simulink model "AttitudeControl"  (R2023a)
settings: Solver=VariableStepAuto  StartTime=0.0  StopTime=10.0  RelTol=1e-3
settings Model: Creator=aan18022  LastModifiedBy=aan18022

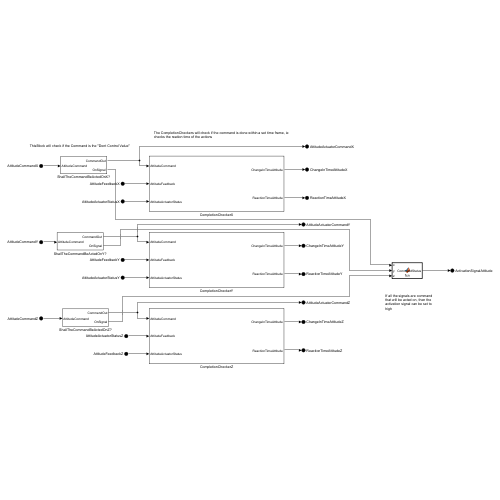
[thumbnail: Simulink's stored preview of the top-level diagram]
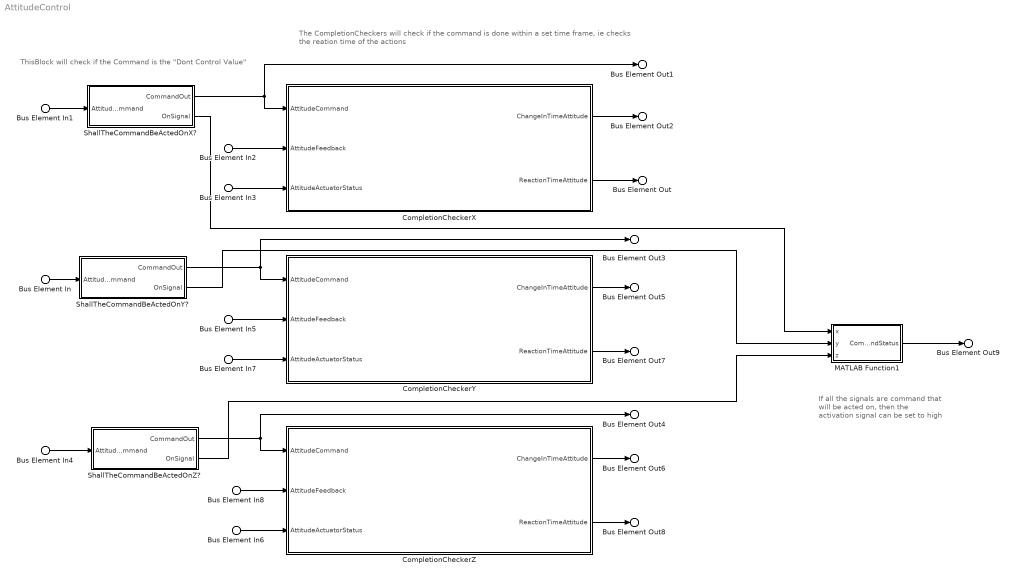
== system AttitudeControl ==
  note: If all the signals are command that will be acted on, then the activation signal can be set to high
  note: The CompletionCheckers will check if the command is done within a set time frame, ie checks the reation time of the actions
  note: ThisBlock will check if the Command is the "Dont Control Value"
  Bus Element In1 : Inport  PortName=AttitudeCommandX
  Bus Element In2 : Inport  Port=2  PortName=AttitudeFeedbackX
  Bus Element In3 : Inport  Port=3  PortName=AttitudeActuatorStatusX
  Bus Element In : Inport  Port=4  PortName=AttitudeCommandY
  Bus Element In4 : Inport  Port=5  PortName=AttitudeCommandZ
  Bus Element In5 : Inport  Port=6  PortName=AttitudeFeedbackY
  Bus Element In6 : Inport  Port=7  PortName=AttitudeFeedbackZ
  Bus Element In7 : Inport  Port=8  PortName=AttitudeActuatorStatusY
  Bus Element In8 : Inport  Port=9  PortName=AttitudeActuatorStatusZ
  CompletionCheckerX : Subsystem
  CompletionCheckerY : Subsystem
  CompletionCheckerZ : Subsystem
  MATLAB Function1 : MATLAB Function  TreatAsAtomicUnit=on
  ShallTheCommandBeActedOnX? : Subsystem
  ShallTheCommandBeActedOnY? : Subsystem
  ShallTheCommandBeActedOnZ? : Subsystem
  Bus Element Out1 : Outport  PortName=AttitudeActuatorCommandX
  Bus Element Out2 : Outport  Port=2  PortName=ChangeInTimeAttitudeX
  Bus Element Out : Outport  Port=3  PortName=ReactionTimeAttitudeX
  Bus Element Out3 : Outport  Port=4  PortName=AttitudeActuatorCommandY
  Bus Element Out4 : Outport  Port=5  PortName=AttitudeActuatorCommandZ
  Bus Element Out5 : Outport  Port=6  PortName=ChangeInTimeAttitudeY
  Bus Element Out6 : Outport  Port=7  PortName=ChangeInTimeAttitudeZ
  Bus Element Out7 : Outport  Port=8  PortName=ReactionTimeAttitudeY
  Bus Element Out8 : Outport  Port=9  PortName=ReactionTimeAttitudeZ
  Bus Element Out9 : Outport  Port=10  PortName=ActivationSignalAttitude
  wires:
  Bus Element In1/1 -> ShallTheCommandBeActedOnX?/1(AttitudeCommand)
  CompletionCheckerY/1(ChangeInTimeAttitude) -> Bus Element Out5/1
  CompletionCheckerY/2(ReactionTimeAttitude) -> Bus Element Out7/1
  Bus Element In2/1 -> CompletionCheckerX/2(AttitudeFeedback)
  Bus Element In8/1 -> CompletionCheckerZ/2(AttitudeFeedback)
  CompletionCheckerZ/2(ReactionTimeAttitude) -> Bus Element Out8/1
  CompletionCheckerX/2(ReactionTimeAttitude) -> Bus Element Out/1
  Bus Element In5/1 -> CompletionCheckerY/2(AttitudeFeedback)
  Bus Element In/1 -> ShallTheCommandBeActedOnY?/1(AttitudeCommand)
  Bus Element In6/1 -> CompletionCheckerZ/3(AttitudeActuatorStatus)
  Bus Element In3/1 -> CompletionCheckerX/3(AttitudeActuatorStatus)
  CompletionCheckerX/1(ChangeInTimeAttitude) -> Bus Element Out2/1
  CompletionCheckerZ/1(ChangeInTimeAttitude) -> Bus Element Out6/1
  Bus Element In4/1 -> ShallTheCommandBeActedOnZ?/1(AttitudeCommand)
  ShallTheCommandBeActedOnX?/1(CommandOut) -> CompletionCheckerX/1(AttitudeCommand), Bus Element Out1/1
  ShallTheCommandBeActedOnY?/1(CommandOut) -> CompletionCheckerY/1(AttitudeCommand), Bus Element Out3/1
  ShallTheCommandBeActedOnZ?/1(CommandOut) -> CompletionCheckerZ/1(AttitudeCommand), Bus Element Out4/1
  Bus Element In7/1 -> CompletionCheckerY/3(AttitudeActuatorStatus)
  ShallTheCommandBeActedOnX?/2(OnSignal) -> MATLAB Function1/1(x)
  ShallTheCommandBeActedOnY?/2(OnSignal) -> MATLAB Function1/2(y)
  ShallTheCommandBeActedOnZ?/2(OnSignal) -> MATLAB Function1/3(z)
  MATLAB Function1/1(CommandStatus) -> Bus Element Out9/1

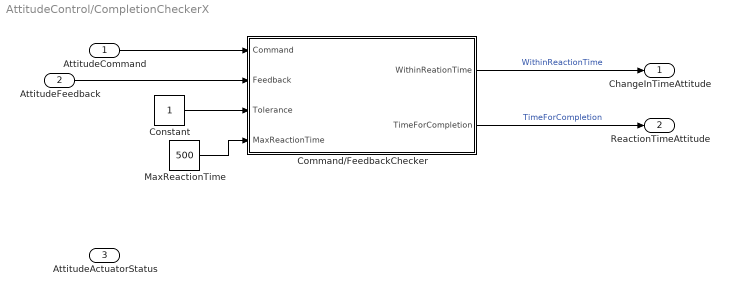
== system AttitudeControl/CompletionCheckerX ==
  AttitudeCommand : Inport
  AttitudeFeedback : Inport  Port=2
  AttitudeActuatorStatus : Inport  Port=3
  Command/FeedbackChecker : Subsystem
  Constant : Constant
  MaxReactionTime : Constant  Value=500
  ChangeInTimeAttitude : Outport
  ReactionTimeAttitude : Outport  Port=2
  wires:
  AttitudeCommand/1 -> Command/FeedbackChecker/1(Command)
  AttitudeFeedback/1 -> Command/FeedbackChecker/2(Feedback)
  Constant/1 -> Command/FeedbackChecker/3(Tolerance)
  Command/FeedbackChecker/1(WithinReationTime) -> ChangeInTimeAttitude/1  "WithinReactionTime"
  Command/FeedbackChecker/2(TimeForCompletion) -> ReactionTimeAttitude/1  "TimeForCompletion"
  MaxReactionTime/1 -> Command/FeedbackChecker/4(MaxReactionTime)

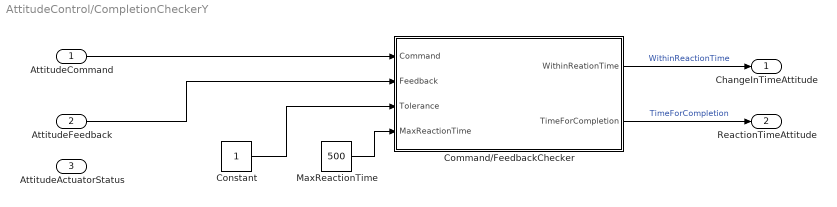
== system AttitudeControl/CompletionCheckerY ==
  AttitudeCommand : Inport
  AttitudeFeedback : Inport  Port=2
  AttitudeActuatorStatus : Inport  Port=3
  Command/FeedbackChecker : Subsystem
  Constant : Constant
  MaxReactionTime : Constant  Value=500
  ChangeInTimeAttitude : Outport
  ReactionTimeAttitude : Outport  Port=2
  wires:
  AttitudeCommand/1 -> Command/FeedbackChecker/1(Command)
  AttitudeFeedback/1 -> Command/FeedbackChecker/2(Feedback)
  Constant/1 -> Command/FeedbackChecker/3(Tolerance)
  Command/FeedbackChecker/1(WithinReationTime) -> ChangeInTimeAttitude/1  "WithinReactionTime"
  Command/FeedbackChecker/2(TimeForCompletion) -> ReactionTimeAttitude/1  "TimeForCompletion"
  MaxReactionTime/1 -> Command/FeedbackChecker/4(MaxReactionTime)

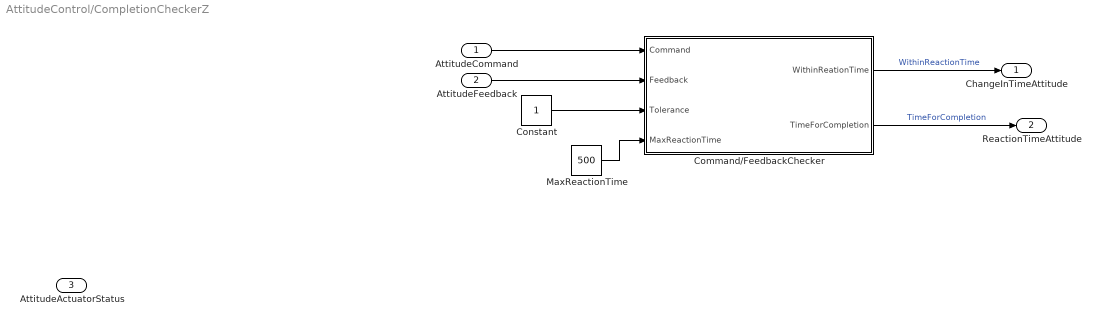
== system AttitudeControl/CompletionCheckerZ ==
  AttitudeCommand : Inport
  AttitudeFeedback : Inport  Port=2
  AttitudeActuatorStatus : Inport  Port=3
  Command/FeedbackChecker : Subsystem
  Constant : Constant
  MaxReactionTime : Constant  Value=500
  ChangeInTimeAttitude : Outport
  ReactionTimeAttitude : Outport  Port=2
  wires:
  AttitudeCommand/1 -> Command/FeedbackChecker/1(Command)
  AttitudeFeedback/1 -> Command/FeedbackChecker/2(Feedback)
  Constant/1 -> Command/FeedbackChecker/3(Tolerance)
  Command/FeedbackChecker/1(WithinReationTime) -> ChangeInTimeAttitude/1  "WithinReactionTime"
  Command/FeedbackChecker/2(TimeForCompletion) -> ReactionTimeAttitude/1  "TimeForCompletion"
  MaxReactionTime/1 -> Command/FeedbackChecker/4(MaxReactionTime)

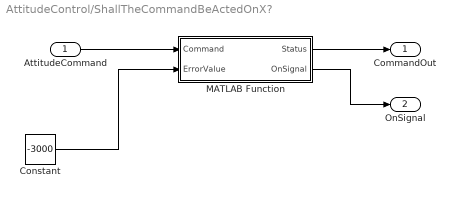
== system AttitudeControl/ShallTheCommandBeActedOnX? ==
  AttitudeCommand : Inport
  Constant : Constant  Value=-3000
  MATLAB Function : MATLAB Function  TreatAsAtomicUnit=on
  CommandOut : Outport
  OnSignal : Outport  Port=2
  wires:
  Constant/1 -> MATLAB Function/2(ErrorValue)
  AttitudeCommand/1 -> MATLAB Function/1(Command)
  MATLAB Function/1(Status) -> CommandOut/1
  MATLAB Function/2(OnSignal) -> OnSignal/1

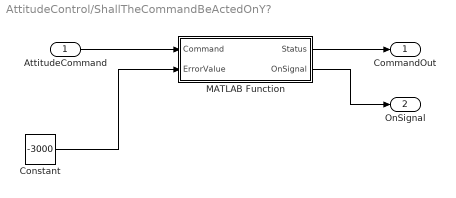
== system AttitudeControl/ShallTheCommandBeActedOnY? ==
  AttitudeCommand : Inport
  Constant : Constant  Value=-3000
  MATLAB Function : MATLAB Function  TreatAsAtomicUnit=on
  CommandOut : Outport
  OnSignal : Outport  Port=2
  wires:
  Constant/1 -> MATLAB Function/2(ErrorValue)
  AttitudeCommand/1 -> MATLAB Function/1(Command)
  MATLAB Function/1(Status) -> CommandOut/1
  MATLAB Function/2(OnSignal) -> OnSignal/1

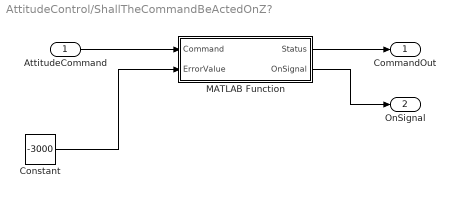
== system AttitudeControl/ShallTheCommandBeActedOnZ? ==
  AttitudeCommand : Inport
  Constant : Constant  Value=-3000
  MATLAB Function : MATLAB Function  TreatAsAtomicUnit=on
  CommandOut : Outport
  OnSignal : Outport  Port=2
  wires:
  Constant/1 -> MATLAB Function/2(ErrorValue)
  AttitudeCommand/1 -> MATLAB Function/1(Command)
  MATLAB Function/1(Status) -> CommandOut/1
  MATLAB Function/2(OnSignal) -> OnSignal/1

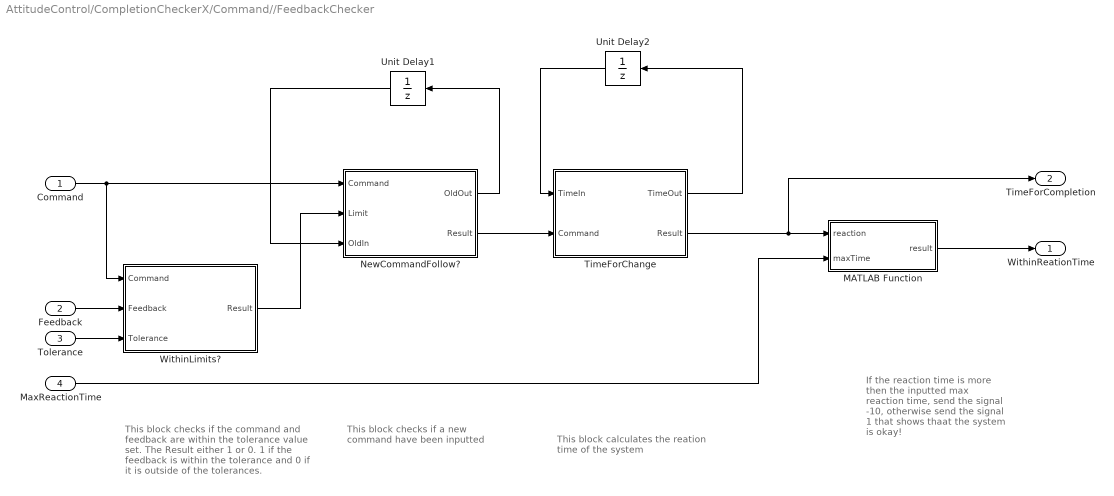
== system AttitudeControl/CompletionCheckerX/Command//FeedbackChecker ==
  note: This block checks if the command and feedback are within the tolerance value set. The Result either 1 or 0. 1 if the feedback is within the tolerance and 0 if it is outside of the tolerances.
  note: This block checks if a new command have been inputted
  note: If the reaction time is more then the inputted max reaction time, send the signal -10, otherwise send the signal 1 that shows thaat the system is okay!
  note: This block calculates the reation time of the system
  Command : Inport
  Feedback : Inport  Port=2
  Tolerance : Inport  Port=3
  MaxReactionTime : Inport  Port=4
  MATLAB Function : MATLAB Function  TreatAsAtomicUnit=on
  NewCommandFollow? : MATLAB Function  TreatAsAtomicUnit=on
  TimeForChange : MATLAB Function  TreatAsAtomicUnit=on
  Unit Delay1 : UnitDelay  InitialCondition=-200  SampleTime=-1  HasFrameUpgradeWarning=on
  Unit Delay2 : UnitDelay  SampleTime=0.5  HasFrameUpgradeWarning=on
  WithinLimits? : MATLAB Function  TreatAsAtomicUnit=on
  WithinReationTime : Outport
  TimeForCompletion : Outport  Port=2
  wires:
  Command/1 -> WithinLimits?/1(Command), NewCommandFollow?/1(Command)
  TimeForChange/1(TimeOut) -> Unit Delay2/1
  NewCommandFollow?/2(Result) -> TimeForChange/2(Command)
  NewCommandFollow?/1(OldOut) -> Unit Delay1/1
  Tolerance/1 -> WithinLimits?/3(Tolerance)
  TimeForChange/2(Result) -> MATLAB Function/1(reaction), TimeForCompletion/1
  WithinLimits?/1(Result) -> NewCommandFollow?/2(Limit)
  MaxReactionTime/1 -> MATLAB Function/2(maxTime)
  Unit Delay2/1 -> TimeForChange/1(TimeIn)
  Unit Delay1/1 -> NewCommandFollow?/3(OldIn)
  Feedback/1 -> WithinLimits?/2(Feedback)
  MATLAB Function/1(result) -> WithinReationTime/1

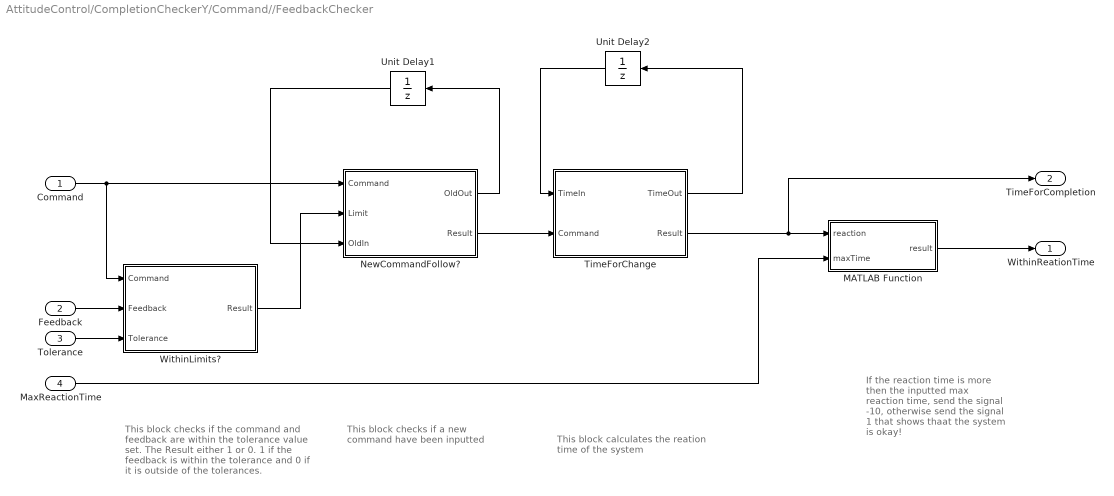
== system AttitudeControl/CompletionCheckerY/Command//FeedbackChecker ==
  note: If the reaction time is more then the inputted max reaction time, send the signal -10, otherwise send the signal 1 that shows thaat the system is okay!
  note: This block checks if the command and feedback are within the tolerance value set. The Result either 1 or 0. 1 if the feedback is within the tolerance and 0 if it is outside of the tolerances.
  note: This block checks if a new command have been inputted
  note: This block calculates the reation time of the system
  Command : Inport
  Feedback : Inport  Port=2
  Tolerance : Inport  Port=3
  MaxReactionTime : Inport  Port=4
  MATLAB Function : MATLAB Function  TreatAsAtomicUnit=on
  NewCommandFollow? : MATLAB Function  TreatAsAtomicUnit=on
  TimeForChange : MATLAB Function  TreatAsAtomicUnit=on
  Unit Delay1 : UnitDelay  InitialCondition=-200  SampleTime=-1  HasFrameUpgradeWarning=on
  Unit Delay2 : UnitDelay  SampleTime=0.5  HasFrameUpgradeWarning=on
  WithinLimits? : MATLAB Function  TreatAsAtomicUnit=on
  WithinReationTime : Outport
  TimeForCompletion : Outport  Port=2
  wires:
  TimeForChange/1(TimeOut) -> Unit Delay2/1
  Command/1 -> WithinLimits?/1(Command), NewCommandFollow?/1(Command)
  Unit Delay2/1 -> TimeForChange/1(TimeIn)
  WithinLimits?/1(Result) -> NewCommandFollow?/2(Limit)
  NewCommandFollow?/1(OldOut) -> Unit Delay1/1
  NewCommandFollow?/2(Result) -> TimeForChange/2(Command)
  MATLAB Function/1(result) -> WithinReationTime/1
  Feedback/1 -> WithinLimits?/2(Feedback)
  Unit Delay1/1 -> NewCommandFollow?/3(OldIn)
  Tolerance/1 -> WithinLimits?/3(Tolerance)
  TimeForChange/2(Result) -> MATLAB Function/1(reaction), TimeForCompletion/1
  MaxReactionTime/1 -> MATLAB Function/2(maxTime)

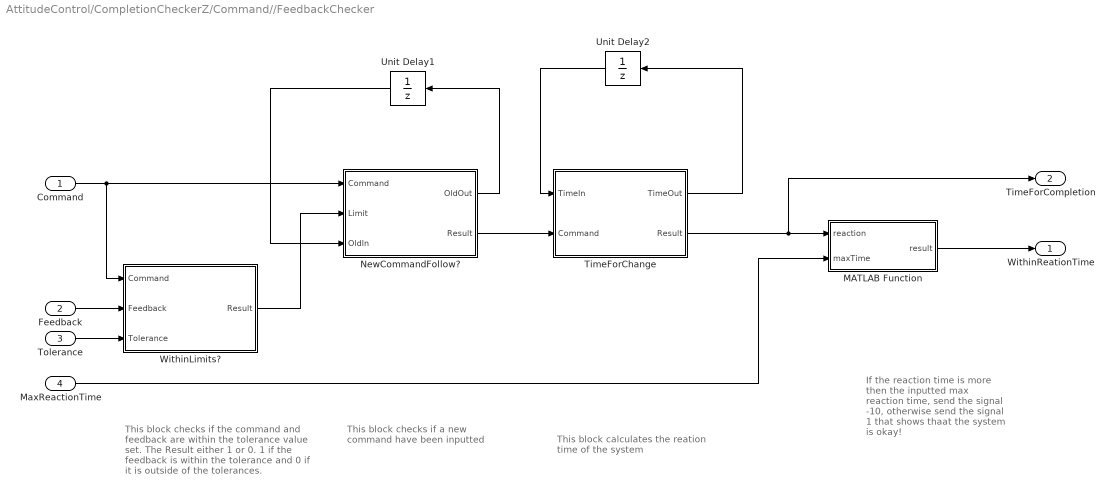
== system AttitudeControl/CompletionCheckerZ/Command//FeedbackChecker ==
  note: This block checks if the command and feedback are within the tolerance value set. The Result either 1 or 0. 1 if the feedback is within the tolerance and 0 if it is outside of the tolerances.
  note: This block checks if a new command have been inputted
  note: If the reaction time is more then the inputted max reaction time, send the signal -10, otherwise send the signal 1 that shows thaat the system is okay!
  note: This block calculates the reation time of the system
  Command : Inport
  Feedback : Inport  Port=2
  Tolerance : Inport  Port=3
  MaxReactionTime : Inport  Port=4
  MATLAB Function : MATLAB Function  TreatAsAtomicUnit=on
  NewCommandFollow? : MATLAB Function  TreatAsAtomicUnit=on
  TimeForChange : MATLAB Function  TreatAsAtomicUnit=on
  Unit Delay1 : UnitDelay  InitialCondition=-200  SampleTime=-1  HasFrameUpgradeWarning=on
  Unit Delay2 : UnitDelay  SampleTime=0.5  HasFrameUpgradeWarning=on
  WithinLimits? : MATLAB Function  TreatAsAtomicUnit=on
  WithinReationTime : Outport
  TimeForCompletion : Outport  Port=2
  wires:
  Command/1 -> WithinLimits?/1(Command), NewCommandFollow?/1(Command)
  TimeForChange/1(TimeOut) -> Unit Delay2/1
  NewCommandFollow?/2(Result) -> TimeForChange/2(Command)
  NewCommandFollow?/1(OldOut) -> Unit Delay1/1
  Tolerance/1 -> WithinLimits?/3(Tolerance)
  TimeForChange/2(Result) -> MATLAB Function/1(reaction), TimeForCompletion/1
  WithinLimits?/1(Result) -> NewCommandFollow?/2(Limit)
  MaxReactionTime/1 -> MATLAB Function/2(maxTime)
  Unit Delay2/1 -> TimeForChange/1(TimeIn)
  Unit Delay1/1 -> NewCommandFollow?/3(OldIn)
  Feedback/1 -> WithinLimits?/2(Feedback)
  MATLAB Function/1(result) -> WithinReationTime/1

== matlab function AttitudeControl/ShallTheCommandBeActedOnY?/MATLAB Function ==
  data: Command input; Status output; OnSignal output; ErrorValue input
function [Status,OnSignal]= fcn(Command,ErrorValue)

if Command == 5000
    Status = 0;
    OnSignal = 0;
elseif Command == ErrorValue
    Status = 0;
    OnSignal = 0;
else
    Status = Command;
    OnSignal = 1;
end

== matlab function AttitudeControl/ShallTheCommandBeActedOnZ?/MATLAB Function ==
  data: Command input; Status output; OnSignal output; ErrorValue input
function [Status,OnSignal]= fcn(Command,ErrorValue)

if Command == 5000
    Status = 0;
    OnSignal = 0;
elseif Command == ErrorValue
    Status = 0;
    OnSignal = 0;
else
    Status = Command;
    OnSignal = 1;
end

== matlab function AttitudeControl/MATLAB Function1 ==
  data: x input; CommandStatus output; y input; z input
function CommandStatus = fcn(x,y,z)

if (x == 1 && y == 1 && z == 1)
    CommandStatus = 1;
else
    CommandStatus = 0;
end

== matlab function AttitudeControl/CompletionCheckerY/Command//FeedbackChecker/MATLAB Function ==
  data: reaction input; maxTime input; result output
function result = fcn(reaction, maxTime)

if reaction <= maxTime
    result = 1;
else
    result =-10;
end

== matlab function AttitudeControl/CompletionCheckerX/Command//FeedbackChecker/MATLAB Function ==
  data: reaction input; maxTime input; result output
function result = fcn(reaction, maxTime)

if reaction <= maxTime
    result = 1;
else
    result =-10;
end

== matlab function AttitudeControl/CompletionCheckerX/Command//FeedbackChecker/WithinLimits? ==
  data: Command input; Feedback input; Tolerance input; Result output
function Result = fcn(Command,Feedback,Tolerance)

upperLimit = Command + Tolerance;
lowerLimit = Command - Tolerance;

if (Feedback >= lowerLimit && Feedback <= upperLimit)
        Result = 1;
else
        Result = 0;
end

== matlab function AttitudeControl/CompletionCheckerZ/Command//FeedbackChecker/WithinLimits? ==
  data: Command input; Feedback input; Tolerance input; Result output
function Result = fcn(Command,Feedback,Tolerance)

upperLimit = Command + Tolerance;
lowerLimit = Command - Tolerance;

if (Feedback >= lowerLimit && Feedback <= upperLimit)
        Result = 1;
else
        Result = 0;
end

== matlab function AttitudeControl/CompletionCheckerX/Command//FeedbackChecker/NewCommandFollow? ==
  data: OldOut output; Command input; Limit input; Result output; OldIn input
function [OldOut,Result]= fcn(Command,Limit,OldIn)

if OldIn == -200
    OldOut = 0;
    Result = 0;
elseif (Limit == 1)
    Result = 1;
    OldOut = Command; 
else
    Result = 0;
    OldOut = OldIn;

end

== matlab function AttitudeControl/CompletionCheckerY/Command//FeedbackChecker/NewCommandFollow? ==
  data: OldOut output; Command input; Limit input; Result output; OldIn input
function [OldOut,Result]= fcn(Command,Limit,OldIn)

if OldIn == -200
    OldOut = 0;
    Result = 0;
elseif (Limit == 1)
    Result = 1;
    OldOut = Command; 
else
    Result = 0;
    OldOut = OldIn;

end

== matlab function AttitudeControl/CompletionCheckerX/Command//FeedbackChecker/TimeForChange ==
  data: TimeIn input; TimeOut output; Command input; Result output
function [TimeOut,Result]= fcn(TimeIn, Command)

if Command == 1
    TimeOut = 0;
    Result = TimeIn;
else
    TimeOut = TimeIn+1;
    Result = 0;
end

== matlab function AttitudeControl/CompletionCheckerY/Command//FeedbackChecker/TimeForChange ==
  data: TimeIn input; TimeOut output; Command input; Result output
function [TimeOut,Result]= fcn(TimeIn, Command)

if Command == 1
    TimeOut = 0;
    Result = TimeIn;
else
    TimeOut = TimeIn+1;
    Result = 0;
end

== matlab function AttitudeControl/CompletionCheckerY/Command//FeedbackChecker/WithinLimits? ==
  data: Command input; Feedback input; Tolerance input; Result output
function Result = fcn(Command,Feedback,Tolerance)

upperLimit = Command + Tolerance;
lowerLimit = Command - Tolerance;

if (Feedback >= lowerLimit && Feedback <= upperLimit)
        Result = 1;
else
        Result = 0;
end

== matlab function AttitudeControl/CompletionCheckerZ/Command//FeedbackChecker/MATLAB Function ==
  data: reaction input; maxTime input; result output
function result = fcn(reaction, maxTime)

if reaction <= maxTime
    result = 1;
else
    result =-10;
end

== matlab function AttitudeControl/CompletionCheckerZ/Command//FeedbackChecker/NewCommandFollow? ==
  data: OldOut output; Command input; Limit input; Result output; OldIn input
function [OldOut,Result]= fcn(Command,Limit,OldIn)

if OldIn == -200
    OldOut = 0;
    Result = 0;
elseif (Limit == 1)
    Result = 1;
    OldOut = Command; 
else
    Result = 0;
    OldOut = OldIn;

end

== matlab function AttitudeControl/CompletionCheckerZ/Command//FeedbackChecker/TimeForChange ==
  data: TimeIn input; TimeOut output; Command input; Result output
function [TimeOut,Result]= fcn(TimeIn, Command)

if Command == 1
    TimeOut = 0;
    Result = TimeIn;
else
    TimeOut = TimeIn+1;
    Result = 0;
end

== matlab function AttitudeControl/ShallTheCommandBeActedOnX?/MATLAB Function ==
  data: Command input; Status output; OnSignal output; ErrorValue input
function [Status,OnSignal]= fcn(Command,ErrorValue)

if Command == 5000
    Status = 0;
    OnSignal = 0;
elseif Command == ErrorValue
    Status = 0;
    OnSignal = 0;
else
    Status = Command;
    OnSignal = 1;
end
